simulink model "exp5_6"  (Simulink 3.00)
settings: Solver=ode45  StartTime=0.0  StopTime=10.0  RelTol=1e-3

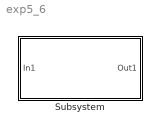
== system exp5_6 ==
  Subsystem : Subsystem

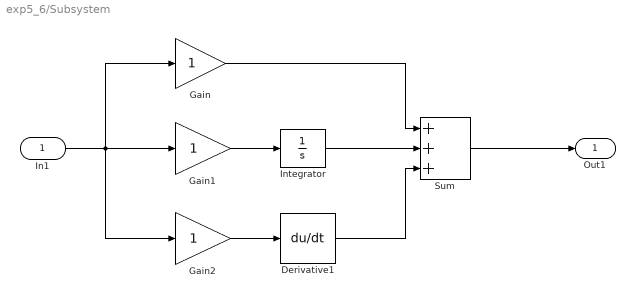
== system exp5_6/Subsystem ==
  In1 : Inport  Port=1  PortWidth=-1  SampleTime=-1  DataType=auto
      settings: SignalType=auto
  Derivative1 : Derivative
  Gain : Gain  Gain=1  SaturateOnIntegerOverflow=on
  Gain1 : Gain  Gain=1  SaturateOnIntegerOverflow=on
  Gain2 : Gain  Gain=1  SaturateOnIntegerOverflow=on
  Integrator : Integrator  ExternalReset=none  InitialConditionSource=internal  InitialCondition=0  LimitOutput=off  UpperSaturationLimit=inf  LowerSaturationLimit=-inf  ShowSaturationPort=off  ShowStatePort=off  AbsoluteTolerance=auto
  Sum : Sum  Inputs=+++  SaturateOnIntegerOverflow=on
  Out1 : Outport  Port=1
  wires:
  Gain1/1 -> Integrator/1
  Gain2/1 -> Derivative1/1
  Gain/1 -> Sum/1
  Integrator/1 -> Sum/2
  Derivative1/1 -> Sum/3
  Sum/1 -> Out1/1
  In1/1 -> Gain1/1, Gain/1, Gain2/1
